simulink model "manual_steer_19b"  (R2019b)
settings: Solver=ode4  StartTime=0.0  StopTime=100  RelTol=1e-3
model workspace (MAT data in the model file):
  x2xx = 0
values from neighbouring files (symbols this model uses):
  KDspd = 0    [time_validation.m]
  KIspd = 0    [time_validation.m]
  KPspd = 20    [time_validation.m]
  PARSa = [ ... (first row only)    [Q_ART_par.m]
  PARSu = zeros(Nu,5)    [Q_ART_par.m]
  TOTALMASS = sum (M,'all')    [Q_ART_par.m]
  v_ref = vconst    (= 5.55555555556)    [time_validation.m]
undefined symbols (not defined in the file or in its folder): axle_rate_limit, BRAKE, brake_lag, brake_rate, DRIVE, Lspd, Nspd, Q0, QD0, RW, Tb, Tmc, Tst, Uspd
libraries: CarMaker4SL x72, simulink x5, TruckMaker4SL x1
(part 2 of 5)

== system manual_steer_19b/truckmaker model/TruckMaker/IPG Vehicle/AFGc ==
  note: steering ratio
  Clock : Clock
  Constant2 : Constant  Value=v_ref
  Constant3 : Constant  Value=PARSa
  From Workspace : FromWorkspace  VariableName=[tstr_in,str_in]  SampleTime=-1
  Gain1 : Gain  Gain=1/20
  MATLAB Function : MATLAB Function  TreatAsAtomicUnit=on
  Rate Limiter1 : RateLimiter  RisingSlewLimit=axle_rate_limit  FallingSlewLimit=-axle_rate_limit  SampleTimeMode=inherited
  To Workspace1 : ToWorkspace  VariableName=time  SampleTime=-1
  brake and drive controller : Subsystem
  find_vx : MATLAB Function  TreatAsAtomicUnit=on
  proc : Subsystem
  q&qd builder : Subsystem
  speed controller : Subsystem
  steering controller : Subsystem
  tractor brake : Outport
  wires:
  speed controller/1(accel command) -> brake and drive controller/1(acc command)
  brake and drive controller/1(tractor brake) -> tractor brake/1
  Rate Limiter1/1 -> steering controller/1(steer6)
  Constant3/1 -> MATLAB Function/2(PARSa)
  Gain1/1 -> MATLAB Function/1(str1)
  MATLAB Function/1(y) -> Rate Limiter1/1
  From Workspace/1 -> Gain1/1
  [q_truckmaker] -> find_vx/1(q)
  find_vx/1(vx6) -> speed controller/2(vxa)
  [qd_truckmaker] -> find_vx/2(qd)
  Constant2/1 -> speed controller/1(speed ref)
  Clock/1 -> To Workspace1/1

== system manual_steer_19b/truckmaker model/TruckMaker/IPG Vehicle/Brake ==
  note: <Your model here>
  note: When replacing the entire braking system,
      | be sure to disable the IPG brake model by using the brake
      | model 'Model Manager off' in the vehicle GUI.
  Sync_In : Inport
  Brake.IF.In : Inport  Port=2
  VhclCtrl.Brake : Inport  Port=3
  tractor brake : Inport  Port=4
  Brake : S-Function  FunctionName=TM_Sfun  Parameters='Brake'  SFunctionDeploymentMode=off  EnableBusSupport=off
  BrakeUpd : S-Function  FunctionName=TM_Sfun  Parameters='BrakeUpd'  SFunctionDeploymentMode=off  EnableBusSupport=off
  BusCreator : BusCreator  Inputs=32
  CreateBus Vhcl.Wheel.PT : Subsystem
  Demux : Demux  Outputs=32
      settings: DisplayOption=none
  Demux1 : Demux  Outputs=3
  Terminator{,1..5} (6 alike) : Terminator
  Sync_Out : Outport
  Vhcl.Wheel.PT : Outport  Port=2
  wires:
  Demux/32 -> BusCreator/32  "Brake IF Trq_DriveSrc_trg d7"
  Demux/31 -> BusCreator/31  "Brake IF Trq_DriveSrc_trg d6"
  Demux/30 -> BusCreator/30  "Brake IF Trq_DriveSrc_trg d5"
  Demux/29 -> BusCreator/29  "Brake IF Trq_DriveSrc_trg d4"
  Demux/28 -> BusCreator/28  "Brake IF Trq_DriveSrc_trg d3"
  Demux/27 -> BusCreator/27  "Brake IF Trq_DriveSrc_trg d2"
  Demux/26 -> BusCreator/26  "Brake IF Trq_DriveSrc_trg d1"
  Demux/25 -> BusCreator/25  "Brake IF Trq_DriveSrc_trg d0"
  Demux/24 -> BusCreator/24  "Brake IF Trq_Reg_trg FR2"
  Demux/23 -> BusCreator/23  "Brake IF Trq_Reg_trg FL2"
  Demux/22 -> BusCreator/22  "Brake IF Trq_Reg_trg RR2"
  Demux/21 -> BusCreator/21  "Brake IF Trq_Reg_trg RL2"
  Demux/20 -> BusCreator/20  "Brake IF Trq_Reg_trg RR"
  Demux/19 -> BusCreator/19  "Brake IF Trq_Reg_trg RL"
  Demux/18 -> BusCreator/18  "Brake IF Trq_Reg_trg FR"
  Demux/17 -> BusCreator/17  "Brake IF Trq_Reg_trg FL"
  Demux/16 -> BusCreator/16  "Brake IF Trq_PB FR2"
  Demux/15 -> BusCreator/15  "Brake IF Trq_PB FL2"
  Demux/14 -> BusCreator/14  "Brake IF Trq_PB RR2"
  Demux/13 -> BusCreator/13  "Brake IF Trq_PB RL2"
  Demux/12 -> BusCreator/12  "Brake IF Trq_PB RR"
  Demux/11 -> BusCreator/11  "Brake IF Trq_PB RL"
  Demux/10 -> BusCreator/10  "Brake IF Trq_PB FR"
  Demux/9 -> BusCreator/9  "Brake IF Trq_PB FL"
  Demux/8 -> BusCreator/8  "Brake IF Trq_WB FR2"
  Demux/7 -> BusCreator/7  "Brake IF Trq_WB FL2"
  BusCreator/1 -> BrakeUpd/2
  Brake/2 -> Demux/1
  BrakeUpd/1 -> Sync_Out/1
  Brake/1 -> BrakeUpd/1  "Sync"
  Brake.IF.In/1 -> Brake/2
  VhclCtrl.Brake/1 -> Brake/3
  Sync_In/1 -> Brake/1
  BrakeUpd/2 -> CreateBus Vhcl.Wheel.PT/1(In)
  CreateBus Vhcl.Wheel.PT/1(Out) -> Vhcl.Wheel.PT/1
  Demux1/2 -> BusCreator/3, BusCreator/4
  Demux1/1 -> BusCreator/1, BusCreator/2
  tractor brake/1 -> Demux1/1
  Demux/4 -> Terminator3/1  "Brake IF Trq_WB RR"
  Demux/3 -> Terminator2/1  "Brake IF Trq_WB RL"
  Demux/2 -> Terminator1/1  "Brake IF Trq_WB FR"
  Demux/1 -> Terminator/1  "Brake IF Trq_WB FL"
  Demux/5 -> Terminator4/1  "Brake IF Trq_WB RL2"
  Demux/6 -> Terminator5/1  "Brake IF Trq_WB RR2"
  Demux1/3 -> BusCreator/5, BusCreator/6

== system manual_steer_19b/truckmaker model/TruckMaker/IPG Vehicle/CarAndTrailer ==
  Sync_In : Inport
  VhclCtrl.Steering : Inport  Port=2
  Vhcl.Wheel.In : Inport  Port=3
  Vhcl.Misc : Inport  Port=4
  CarAndTrailerUpd : Subsystem
  Forces : Subsystem
  Ground : Ground
  Kinematics : Subsystem
  Kinetics : Subsystem
  Steering : Subsystem
  Terminator : Terminator
  Terminator1 : Terminator
  Trailer : Subsystem
  Sync_Out : Outport
  Brake.IF.In : Outport  Port=2
  wires:
  Ground/1 -> CarAndTrailerUpd/14(Vhcl.Fr1A)
  Trailer/13(Car.Hitch.FrcTrq) -> CarAndTrailerUpd/13(Car.Hitch.FrcTrq)
  Trailer/12(Vhcl.Wheel.FR2) -> CarAndTrailerUpd/12(Vhcl.Wheel.FR2)
  Trailer/11(Vhcl.Wheel.FL2) -> CarAndTrailerUpd/11(Vhcl.Wheel.FL2)
  Trailer/10(Vhcl.Wheel.RR2) -> CarAndTrailerUpd/10(Vhcl.Wheel.RR2)
  Trailer/9(Vhcl.Wheel.RL2) -> CarAndTrailerUpd/9(Vhcl.Wheel.RL2)
  Trailer/8(Vhcl.Wheel.RR) -> CarAndTrailerUpd/8(Vhcl.Wheel.RR)
  Trailer/7(Vhcl.Wheel.RL) -> CarAndTrailerUpd/7(Vhcl.Wheel.RL)
  Trailer/6(Vhcl.Wheel.FR) -> CarAndTrailerUpd/6(Vhcl.Wheel.FR)
  Trailer/5(Vhcl.Wheel.FL) -> CarAndTrailerUpd/5(Vhcl.Wheel.FL)
  Trailer/4(Vhcl.PoI) -> CarAndTrailerUpd/4(Vhcl.PoI)
  Trailer/3(Vhcl.Motion) -> CarAndTrailerUpd/3(Vhcl.Motion)
  Trailer/2(Vhcl.Steering) -> CarAndTrailerUpd/2(Vhcl.Steering)
  Trailer/1(Sync_Out) -> CarAndTrailerUpd/1(Sync_In)
  CarAndTrailerUpd/2(Brake.IF.In) -> Brake.IF.In/1
  Vhcl.Misc/1 -> Terminator1/1
  Vhcl.Wheel.In/1 -> Terminator/1
  Kinetics/6(WheelCarrier.Misc) -> Trailer/6(WheelCarrier.Misc)
  Kinetics/5(Car.Trq_T2W) -> Trailer/5(Car.Trq_T2W)
  Steering/2(Steer.IF) -> Kinematics/2(Steer.IF)
  Kinetics/4(Car.Fr1) -> Trailer/4(Car.Fr1)
  Kinetics/3(Car.Hitch) -> Trailer/3(Car.Hitch)
  Kinetics/2(Trailer.Load) -> Trailer/2(Trailer.Load)
  VhclCtrl.Steering/1 -> Steering/2(VhclCtrl.Steering)
  Sync_In/1 -> Steering/1(Sync_In)
  Steering/1(Sync_Out) -> Kinematics/1(Sync_In)
  Kinetics/1(Sync_Out) -> Trailer/1(Sync_In)
  Kinematics/5(lBuf) -> Forces/5(lBuf)
  Forces/8(FBuf_ext) -> Kinetics/8(FBuf_ext)
  Forces/4(Car.Load) -> Kinetics/4(Car.Load)
  Forces/7(FStabi_ext) -> Kinetics/7(FStabi_ext)
  Forces/6(FDamp_ext) -> Kinetics/6(FDamp_ext)
  Forces/5(FSpring_ext) -> Kinetics/5(FSpring_ext)
  Forces/2(Car.Virtual) -> Kinetics/2(Car.Virtual)
  Kinematics/2(lSpring) -> Forces/2(lSpring)
  Kinematics/3(vDamp) -> Forces/3(vDamp)
  Forces/3(Car.Aero) -> Kinetics/3(Car.Aero)
  Forces/1(Sync_Out) -> Kinetics/1(Sync_In)
  Kinematics/1(Sync_Out) -> Forces/1(Sync_In)
  Kinematics/4(lStabi) -> Forces/4(lStabi)
  CarAndTrailerUpd/1(Sync_Out) -> Sync_Out/1

== system manual_steer_19b/truckmaker model/TruckMaker/IPG Vehicle/PowerTrain ==
  note: When replacing the entire powertrain,
      | be sure to disable the IPG powertrain model by using the powertrain
      | model 'Model Manager off' in the vehicle GUI.
  note: <Your model here>
  Sync_In : Inport
  Vhcl.Wheel.PT : Inport  Port=2
  VhclCtrl.PT : Inport  Port=3
  BusCreator : BusCreator  Inputs=70
  Demux : Demux  Outputs=70
      settings: DisplayOption=none
  PowerTrain : S-Function  FunctionName=TM_Sfun  Parameters='PowerTrain'  SFunctionDeploymentMode=off  EnableBusSupport=off
  PowerTrainUpd : S-Function  FunctionName=TM_Sfun  Parameters='PowerTrainUpd'  SFunctionDeploymentMode=off  EnableBusSupport=off
  Sync_Out : Outport
  wires:
  Demux/70 -> BusCreator/70  "PT IF WFR2 Trq_BrakeReg_max"
  Demux/69 -> BusCreator/69  "PT IF WFR2 Trq_BrakeReg"
  Demux/68 -> BusCreator/68  "PT IF WFR2 Trq_Supp2WC"
  Demux/67 -> BusCreator/67  "PT IF WFR2 Trq_Drive"
  Demux/66 -> BusCreator/66  "PT IF WFR2 Trq_B2W"
  Demux/65 -> BusCreator/65  "PT IF WFR2 rotv"
  Demux/64 -> BusCreator/64  "PT IF WFR2 rot"
  Demux/63 -> BusCreator/63  "PT IF WFL2 Trq_BrakeReg_max"
  Demux/62 -> BusCreator/62  "PT IF WFL2 Trq_BrakeReg"
  Demux/59 -> BusCreator/59  "PT IF WFL2 Trq_B2W"
  Demux/58 -> BusCreator/58  "PT IF WFL2 rotv"
  Demux/57 -> BusCreator/57  "PT IF WFL2 rot"
  Demux/56 -> BusCreator/56  "PT IF WRR2 Trq_BrakeReg_max"
  Demux/55 -> BusCreator/55  "PT IF WRR2 Trq_BrakeReg"
  Demux/52 -> BusCreator/52  "PT IF WRR2 Trq_B2W"
  Demux/51 -> BusCreator/51  "PT IF WRR2 rotv"
  Demux/50 -> BusCreator/50  "PT IF WRR2 rot"
  Demux/49 -> BusCreator/49  "PT IF WRL2 Trq_BrakeReg_max"
  Demux/48 -> BusCreator/48  "PT IF WRL2 Trq_BrakeReg"
  Demux/45 -> BusCreator/45  "PT IF WRL2 Trq_B2W"
  Demux/44 -> BusCreator/44  "PT IF WRL2 rotv"
  Demux/43 -> BusCreator/43  "PT IF WRL2 rot"
  Demux/42 -> BusCreator/42  "PT IF WRR Trq_BrakeReg_max"
  Demux/41 -> BusCreator/41  "PT IF WRR Trq_BrakeReg"
  Demux/38 -> BusCreator/38  "PT IF WRR Trq_B2W"
  Demux/37 -> BusCreator/37  "PT IF WRR rotv"
  Demux/36 -> BusCreator/36  "PT IF WRR rot"
  Demux/35 -> BusCreator/35  "PT IF WRL Trq_BrakeReg_max"
  Demux/34 -> BusCreator/34  "PT IF WRL Trq_BrakeReg"
  Demux/31 -> BusCreator/31  "PT IF WRL Trq_B2W"
  Demux/30 -> BusCreator/30  "PT IF WRL rotv"
  Demux/29 -> BusCreator/29  "PT IF WRL rot"
  Demux/28 -> BusCreator/28  "PT IF WFR Trq_BrakeReg_max"
  Demux/27 -> BusCreator/27  "PT IF WFR Trq_BrakeReg"
  Demux/24 -> BusCreator/24  "PT IF WFR Trq_B2W"
  Demux/23 -> BusCreator/23  "PT IF WFR rotv"
  Demux/22 -> BusCreator/22  "PT IF WFR rot"
  Demux/21 -> BusCreator/21  "PT IF WFL Trq_BrakeReg_max"
  Demux/20 -> BusCreator/20  "PT IF WFL Trq_BrakeReg"
  Demux/17 -> BusCreator/17  "PT IF WFL Trq_B2W"
  Demux/16 -> BusCreator/16  "PT IF WFL rotv"
  Demux/15 -> BusCreator/15  "PT IF WFL rot"
  Demux/14 -> BusCreator/14  "PT IF DL_iDiff_mean"
  Demux/13 -> BusCreator/13  "PT IF Trq_Supp2BdyEng y"
  Demux/12 -> BusCreator/12  "PT IF Trq_Supp2BdyEng x"
  Demux/11 -> BusCreator/11  "PT IF Trq_Supp2Bdy1B z"
  Demux/10 -> BusCreator/10  "PT IF Trq_Supp2Bdy1B y"
  Demux/9 -> BusCreator/9  "PT IF Trq_Supp2Bdy1B x"
  Demux/8 -> BusCreator/8  "PT IF Trq_Supp2Bdy1 z"
  Demux/7 -> BusCreator/7  "PT IF Trq_Supp2Bdy1 y"
  Demux/6 -> BusCreator/6  "PT IF Trq_Supp2Bdy1 x"
  Demux/5 -> BusCreator/5  "PT IF Engine_rotv"
  Demux/4 -> BusCreator/4  "PT IF GearNo"
  Demux/3 -> BusCreator/3  "PT IF OperationError"
  Demux/2 -> BusCreator/2  "PT IF OperationState"
  Demux/1 -> BusCreator/1  "PT IF Ignition"
  BusCreator/1 -> PowerTrainUpd/2
  PowerTrain/2 -> Demux/1
  Sync_In/1 -> PowerTrain/1
  PowerTrainUpd/1 -> Sync_Out/1
  PowerTrain/1 -> PowerTrainUpd/1  "Sync"
  VhclCtrl.PT/1 -> PowerTrain/3
  Vhcl.Wheel.PT/1 -> PowerTrain/2
  Demux/60 -> BusCreator/60  "PT IF WFL2 Trq_Drive"
  Demux/61 -> BusCreator/61  "PT IF WFL2 Trq_Supp2WC"
  Demux/18 -> BusCreator/18  "PT IF WFL Trq_Drive"
  Demux/19 -> BusCreator/19  "PT IF WFL Trq_Supp2WC"
  Demux/25 -> BusCreator/25  "PT IF WFR Trq_Drive"
  Demux/26 -> BusCreator/26  "PT IF WFR Trq_Supp2WC"
  Demux/32 -> BusCreator/32  "PT IF WRL Trq_Drive"
  Demux/33 -> BusCreator/33  "PT IF WRL Trq_Supp2WC"
  Demux/39 -> BusCreator/39  "PT IF WRR Trq_Drive"
  Demux/40 -> BusCreator/40  "PT IF WRR Trq_Supp2WC"
  Demux/46 -> BusCreator/46  "PT IF WRL2 Trq_Drive"
  Demux/47 -> BusCreator/47  "PT IF WRL2 Trq_Supp2WC"
  Demux/53 -> BusCreator/53  "PT IF WRR2 Trq_Drive"
  Demux/54 -> BusCreator/54  "PT IF WRR2 Trq_Supp2WC"

== system manual_steer_19b/truckmaker model/TruckMaker/VehicleControl/CreateBus Vhcl.Misc ==
  In1 : Inport
  Bus Creator5 : BusCreator  Inputs=11
  Demux5 : Demux  Outputs=11
      settings: DisplayOption=none
  Out1 : Outport
  wires:
  Demux5/11 -> Bus Creator5/11  "Vhcl Wind_vel_0 z"
  Demux5/10 -> Bus Creator5/10  "Vhcl Wind_vel_0 y"
  Demux5/9 -> Bus Creator5/9  "Vhcl Wind_vel_0 x"
  Demux5/8 -> Bus Creator5/8  "Vhcl DL2BdyEng y"
  Demux5/7 -> Bus Creator5/7  "Vhcl DL2BdyEng x"
  Demux5/6 -> Bus Creator5/6  "Vhcl TrqDL2Bdy1B z"
  Demux5/5 -> Bus Creator5/5  "Vhcl TrqDL2Bdy1B y"
  Demux5/4 -> Bus Creator5/4  "Vhcl TrqDL2Bdy1B x"
  Demux5/3 -> Bus Creator5/3  "Vhcl Trq_DL2Bdy1 z"
  In1/1 -> Demux5/1
  Bus Creator5/1 -> Out1/1
  Demux5/2 -> Bus Creator5/2  "Vhcl Trq_DL2Bdy1 y"
  Demux5/1 -> Bus Creator5/1  "Vhcl Trq_DL2Bdy1 x"

== system manual_steer_19b/truckmaker model/TruckMaker/VehicleControl/CreateBus Vhcl.Wheel.In ==
  In1 : Inport
  Bus Creator1 : BusCreator  Inputs=24
  Demux1 : Demux  Outputs=24
      settings: DisplayOption=none
  Out1 : Outport
  wires:
  Demux1/12 -> Bus Creator1/12  "Vhcl Wheel RR rotv"
  Demux1/11 -> Bus Creator1/11  "Vhcl Wheel RR Trq_DL2WC"
  Demux1/10 -> Bus Creator1/10  "Vhcl Wheel RR Trq_B2WC"
  Demux1/9 -> Bus Creator1/9  "Vhcl Wheel RL rotv"
  Demux1/8 -> Bus Creator1/8  "Vhcl Wheel RL Trq_DL2WC"
  Demux1/7 -> Bus Creator1/7  "Vhcl Wheel RL Trq_B2WC"
  Demux1/6 -> Bus Creator1/6  "Vhcl Wheel FR rotv"
  Demux1/5 -> Bus Creator1/5  "Vhcl Wheel FR Trq_DL2WC"
  Demux1/4 -> Bus Creator1/4  "Vhcl Wheel FR Trq_B2WC"
  Demux1/3 -> Bus Creator1/3  "Vhcl Wheel FL rotv"
  Demux1/2 -> Bus Creator1/2  "Vhcl Wheel FL Trq_DL2WC"
  Demux1/1 -> Bus Creator1/1  "Vhcl Wheel FL Trq_B2WC"
  Bus Creator1/1 -> Out1/1
  In1/1 -> Demux1/1
  Demux1/24 -> Bus Creator1/24  "Vhcl Wheel FR2 rotv"
  Demux1/23 -> Bus Creator1/23  "Vhcl Wheel FR2 Trq_DL2WC"
  Demux1/22 -> Bus Creator1/22  "Vhcl Wheel FR2 Trq_B2WC"
  Demux1/21 -> Bus Creator1/21  "Vhcl Wheel FL2 rotv"
  Demux1/20 -> Bus Creator1/20  "Vhcl Wheel FL2 Trq_DL2WC"
  Demux1/19 -> Bus Creator1/19  "Vhcl Wheel FL2 Trq_B2WC"
  Demux1/18 -> Bus Creator1/18  "Vhcl Wheel RR2 rotv"
  Demux1/17 -> Bus Creator1/17  "Vhcl Wheel RR2 Trq_DL2WC"
  Demux1/16 -> Bus Creator1/16  "Vhcl Wheel RR2 Trq_B2WC"
  Demux1/15 -> Bus Creator1/15  "Vhcl Wheel RL2 rotv"
  Demux1/14 -> Bus Creator1/14  "Vhcl Wheel RL2 Trq_DL2WC"
  Demux1/13 -> Bus Creator1/13  "Vhcl Wheel RL2 Trq_B2WC"

== system manual_steer_19b/truckmaker model/TruckMaker/VehicleControl/CreateBus VhclCtrl ==
  In : Inport
  BusCreator : BusCreator  Inputs=29
  Demux : Demux  Outputs=29
      settings: DisplayOption=none
  Out : Outport
  wires:
  Demux/29 -> BusCreator/29  "VhclCtrl Lights Reverse"
  Demux/28 -> BusCreator/28  "VhclCtrl Lights Brake"
  Demux/27 -> BusCreator/27  "VhclCtrl Lights FogRear"
  Demux/26 -> BusCreator/26  "VhclCtrl Lights FogFrontR"
  Demux/25 -> BusCreator/25  "VhclCtrl Lights FogFrontL"
  Demux/24 -> BusCreator/24  "VhclCtrl Lights IndR"
  Demux/23 -> BusCreator/23  "VhclCtrl Lights IndL"
  Demux/22 -> BusCreator/22  "VhclCtrl Lights ParkR"
  Demux/21 -> BusCreator/21  "VhclCtrl Lights ParkL"
  Demux/20 -> BusCreator/20  "VhclCtrl Lights Daytime"
  Demux/19 -> BusCreator/19  "VhclCtrl Lights HighBeam"
  Demux/18 -> BusCreator/18  "VhclCtrl Lights LowBeam"
  Demux/17 -> BusCreator/17  "VhclCtrl Steering Trq"
  Demux/16 -> BusCreator/16  "VhclCtrl Steering AngAcc"
  Demux/15 -> BusCreator/15  "VhclCtrl Steering AngVel"
  Demux/14 -> BusCreator/14  "VhclCtrl Steering Ang"
  Demux/13 -> BusCreator/13  "VhclCtrl Gas"
  Demux/12 -> BusCreator/12  "VhclCtrl Clutch"
  Demux/11 -> BusCreator/11  "VhclCtrl BrakePark"
  Demux/10 -> BusCreator/10  "VhclCtrl Brake"
  Demux/9 -> BusCreator/9  "VhclCtrl SelectorCtrl"
  Demux/8 -> BusCreator/8  "VhclCtrl GearNo"
  Demux/7 -> BusCreator/7  "VhclCtrl UserSignal4"
  Demux/6 -> BusCreator/6  "VhclCtrl UserSignal3"
  Demux/5 -> BusCreator/5  "VhclCtrl UserSignal2"
  Demux/4 -> BusCreator/4  "VhclCtrl UserSignal1"
  Demux/3 -> BusCreator/3  "VhclCtrl UserSignal0"
  Demux/2 -> BusCreator/2  "VhclCtrl Key"
  Demux/1 -> BusCreator/1  "VhclCtrl SST"
  BusCreator/1 -> Out/1
  In/1 -> Demux/1

== system manual_steer_19b/truckmaker model/TruckMaker/VehicleControl/CreateBus VhclCtrl.PT ==
  In1 : Inport
  BusCreator1 : BusCreator  Inputs=12
  Demux1 : Demux  Outputs=12
      settings: DisplayOption=none
  Out1 : Outport
  wires:
  BusCreator1/1 -> Out1/1
  In1/1 -> Demux1/1
  Demux1/1 -> BusCreator1/1  "VhclCtrl SST"
  Demux1/2 -> BusCreator1/2  "VhclCtrl Key"
  Demux1/3 -> BusCreator1/3  "VhclCtrl UserSignal0"
  Demux1/4 -> BusCreator1/4  "VhclCtrl UserSignal1"
  Demux1/5 -> BusCreator1/5  "VhclCtrl UserSignal2"
  Demux1/6 -> BusCreator1/6  "VhclCtrl UserSignal3"
  Demux1/7 -> BusCreator1/7  "VhclCtrl UserSignal4"
  Demux1/8 -> BusCreator1/8  "VhclCtrl GearNo"
  Demux1/9 -> BusCreator1/9  "VhclCtrl SelectorCtrl"
  Demux1/10 -> BusCreator1/10  "VhclCtrl Clutch"
  Demux1/11 -> BusCreator1/11  "VhclCtrl Gas"
  Demux1/12 -> BusCreator1/12  "VhclCtrl Brake"

== system manual_steer_19b/truckmaker model/TruckMaker/VehicleControl/CreateBus VhclCtrl.Steering ==
  In1 : Inport
  Bus Creator : BusCreator  Inputs=5
  Demux : Demux  Outputs=5
      settings: DisplayOption=none
  Out1 : Outport
  wires:
  In1/1 -> Demux/1
  Bus Creator/1 -> Out1/1
  Demux/1 -> Bus Creator/1  "VhclCtrl Steering Ang"
  Demux/5 -> Bus Creator/5  "VhclCtrl Steering ByTrq"
  Demux/3 -> Bus Creator/3  "VhclCtrl Steering AngAcc"
  Demux/2 -> Bus Creator/2  "VhclCtrl Steering AngVel"
  Demux/4 -> Bus Creator/4  "VhclCtrl Steering Trq"

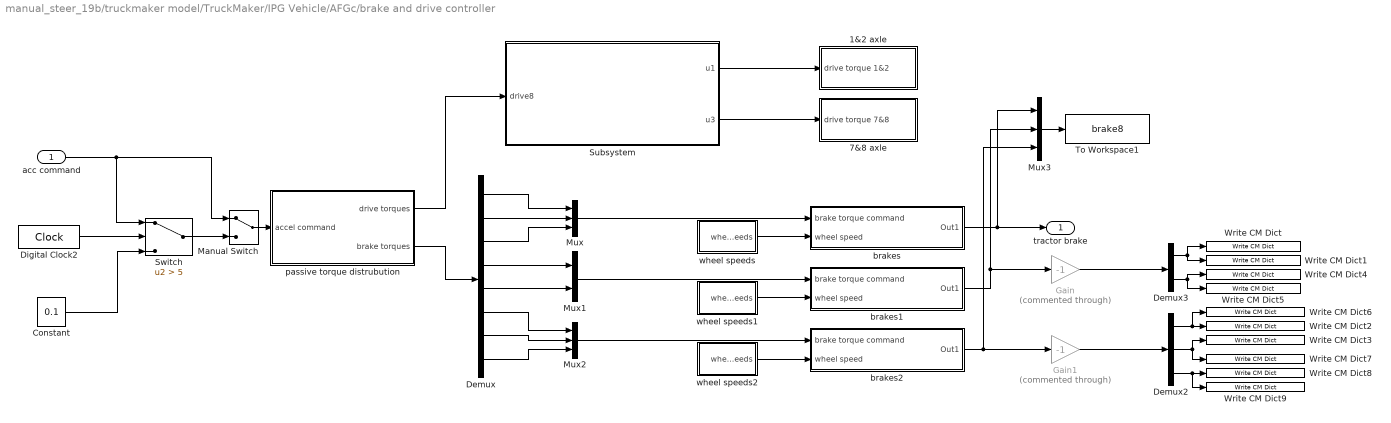
== system manual_steer_19b/truckmaker model/TruckMaker/IPG Vehicle/AFGc/brake and drive controller ==
  acc command : Inport
  1&2 axle : Subsystem
  7&8 axle : Subsystem
  Constant : Constant  Value=0.1
  Demux : Demux  Outputs=8
  Demux2 : Demux  Outputs=3
  Demux3 : Demux  Outputs=2
  Digital Clock2 : DigitalClock  SampleTime=0.001
  Gain : Gain  Commented=through  Gain=-1
  Gain1 : Gain  Commented=through  Gain=-1
  Manual Switch : ManualSwitch
  Mux : Mux  Inputs=3
  Mux1 : Mux  Inputs=2
  Mux2 : Mux  Inputs=3
  Mux3 : Mux  Inputs=3
  Subsystem : Subsystem
  Switch : Switch  Criteria=u2 > Threshold  Threshold=5
  To Workspace1 : ToWorkspace  VariableName=brake8  SampleTime=-1
  Write CM Dict : CarMaker4SL/Write CM Dict  xname=Tr.Brake.Trq_FL_ext  xsync=off
  Write CM Dict1 : CarMaker4SL/Write CM Dict  xname=Tr.Brake.Trq_FR_ext  xsync=off
  Write CM Dict2 : CarMaker4SL/Write CM Dict  xname=Tr2.Brake.Trq_FR_ext  xsync=off
  Write CM Dict3 : CarMaker4SL/Write CM Dict  xname=Tr2.Brake.Trq_ML_ext  xsync=off
  Write CM Dict4 : CarMaker4SL/Write CM Dict  xname=Tr.Brake.Trq_RL_ext  xsync=off
  Write CM Dict5 : CarMaker4SL/Write CM Dict  xname=Tr.Brake.Trq_RR_ext  xsync=off
  Write CM Dict6 : CarMaker4SL/Write CM Dict  xname=Tr2.Brake.Trq_FL_ext  xsync=off
  Write CM Dict7 : CarMaker4SL/Write CM Dict  xname=Tr2.Brake.Trq_MR_ext  xsync=off
  Write CM Dict8 : CarMaker4SL/Write CM Dict  xname=Tr2.Brake.Trq_RL_ext  xsync=off
  Write CM Dict9 : CarMaker4SL/Write CM Dict  xname=Tr2.Brake.Trq_RR_ext  xsync=off
  brakes : Subsystem
  brakes1 : Subsystem
  brakes2 : Subsystem
  passive torque distrubution : Subsystem
  wheel speeds : Subsystem
  wheel speeds1 : Subsystem
  wheel speeds2 : Subsystem
  tractor brake : Outport  VectorParamsAs1DForOutWhenUnconnected=off
  wires:
  passive torque distrubution/2(brake torques) -> Demux/1
  Mux/1 -> brakes/1(brake torque command)
  Mux1/1 -> brakes1/1(brake torque command)
  wheel speeds1/1(wheel speeds) -> brakes1/2(wheel speed)
  Mux2/1 -> brakes2/1(brake torque command)
  brakes/1(Out1) -> tractor brake/1, Mux3/1
  Mux3/1 -> To Workspace1/1
  Subsystem/1(u1) -> 1&2 axle/1(drive torque 1&2)
  Subsystem/2(u3) -> 7&8 axle/1(drive torque 7&8)
  wheel speeds2/1(wheel speeds) -> brakes2/2(wheel speed)
  wheel speeds/1(wheel speeds) -> brakes/2(wheel speed)
  Demux/1 -> Mux/1
  Demux/2 -> Mux/2
  Demux/3 -> Mux/3
  Demux/5 -> Mux1/2
  Demux/4 -> Mux1/1
  Demux/6 -> Mux2/1
  Demux/7 -> Mux2/2
  Demux/8 -> Mux2/3
  brakes1/1(Out1) -> Gain/1, Mux3/2
  Demux3/2 -> Write CM Dict4/1, Write CM Dict5/1
  Demux3/1 -> Write CM Dict/1, Write CM Dict1/1
  brakes2/1(Out1) -> Gain1/1, Mux3/3
  Demux2/1 -> Write CM Dict2/1, Write CM Dict6/1
  Demux2/2 -> Write CM Dict7/1, Write CM Dict3/1
  Demux2/3 -> Write CM Dict9/1, Write CM Dict8/1
  passive torque distrubution/1(drive torques) -> Subsystem/1(drive8)
  Gain/1 -> Demux3/1
  Gain1/1 -> Demux2/1
  acc command/1 -> Switch/1, Manual Switch/1
  Constant/1 -> Switch/3
  Digital Clock2/1 -> Switch/2
  Manual Switch/1 -> passive torque distrubution/1(accel command)
  Switch/1 -> Manual Switch/2

== system manual_steer_19b/truckmaker model/TruckMaker/IPG Vehicle/AFGc/proc ==
  Constant1 : Constant  Value=PARSu
  Constant2 : Constant  Value=PARSa
  MatMaker : MATLAB Function  TreatAsAtomicUnit=on
  To Workspace1 : ToWorkspace  Commented=on  VariableName=Va_out  SampleTime=-1
  To Workspace3 : ToWorkspace  Commented=on  VariableName=Vj_out  SampleTime=-1
  To Workspace5 : ToWorkspace  Commented=on  VariableName=Vg_out  SampleTime=-1
  To Workspace6 : ToWorkspace  VariableName=Vgg_out  SampleTime=-1
  To Workspace7 : ToWorkspace  Commented=on  VariableName=Vaa_out  SampleTime=-1
  wires:
  [qd_truckmaker] -> MatMaker/2(qd)
  MatMaker/1(Va) -> To Workspace1/1
  [q_truckmaker] -> MatMaker/1(q)
  MatMaker/5(Vgg) -> To Workspace6/1
  MatMaker/3(Vj) -> To Workspace3/1
  Constant1/1 -> MatMaker/3(PARSu)
  MatMaker/4(Vg) -> To Workspace5/1
  Constant2/1 -> MatMaker/4(PARSa)
  MatMaker/2(Vaa) -> To Workspace7/1

== system manual_steer_19b/truckmaker model/TruckMaker/IPG Vehicle/AFGc/q&qd builder ==
  Read CM Dict1 : CarMaker4SL/Read CM Dict  xname=Tr.ay  xsync=off  xstime=Continuous
  Read CM Dict2 : CarMaker4SL/Read CM Dict  xname=Tr2.ay  xsync=off  xstime=Continuous
  Read CM Dict3 : CarMaker4SL/Read CM Dict  xname=Car.ay  xsync=off  xstime=Continuous
  To Workspace : ToWorkspace  VariableName=q_out_truckmaker  SampleTime=-1
      settings: Save2DSignal=2-D array (concatenate along first dimension)
  To Workspace1 : ToWorkspace  VariableName=qd_out_truckmaker  SampleTime=-1
      settings: Save2DSignal=2-D array (concatenate along first dimension)
  To Workspace2 : ToWorkspace  VariableName=lat_acc_u1_out  SampleTime=-1
      settings: Save2DSignal=2-D array (concatenate along first dimension)
  To Workspace3 : ToWorkspace  VariableName=lat_acc_u2_out  SampleTime=-1
      settings: Save2DSignal=2-D array (concatenate along first dimension)
  To Workspace4 : ToWorkspace  VariableName=lat_acc_u3_out  SampleTime=-1
      settings: Save2DSignal=2-D array (concatenate along first dimension)
  build q : Subsystem
  build qd : Subsystem
  tag scope: q_truckmaker=global, qd_truckmaker=global
  wires:
  build q/1(q) -> To Workspace/1, [q_truckmaker]
  build qd/1(qd) -> To Workspace1/1, [qd_truckmaker]
  Read CM Dict3/1 -> To Workspace2/1
  Read CM Dict1/1 -> To Workspace3/1
  Read CM Dict2/1 -> To Workspace4/1

== system manual_steer_19b/truckmaker model/TruckMaker/IPG Vehicle/AFGc/speed controller ==
  speed ref : Inport
  vxa : Inport  Port=2
  PID Controller : simulink/Continuous/PID Controller  Controller=PID  Form=Parallel  TimeDomain=Discrete-time  SampleTime=-1  IntegratorMethod=Forward Euler  FilterMethod=Forward Euler  ControllerParametersSource=internal  P=KPspd  I=KIspd  D=KDspd  N=Nspd  UseFilter=on  TunerSelectOption=Transfer Function Based (PID Tuner App)  InitialConditionSource=internal  InitialConditionForIntegrator=0  InitialConditionForFilter=0  DifferentiatorICPrevScaledInput=0  ExternalReset=none  TrackingMode=off  Kt=1  LimitOutput=on  UpperSaturationLimit=Uspd  LowerSaturationLimit=Lspd  LinearizeAsGain=on  AntiWindupMode=clamping  Kb=1  POutMin=[]  POutMax=[]  IOutMin=[]  IOutMax=[]  DOutMin=[]  DOutMax=[]  NOutMin=[]  NOutMax=[]  SumOutMin=[]  SumOutMax=[]  SaturationOutMin=[]  SaturationOutMax=[]  PParamMin=[]  PParamMax=[]  IParamMin=[]  IParamMax=[]  DParamMin=[]  DParamMax=[]  NParamMin=[]  NParamMax=[]  KbParamMin=[]  KbParamMax=[]  KtParamMin=[]  KtParamMax=[]  KbOutMin=[]  KbOutMax=[]  KtOutMin=[]  KtOutMax=[]  IntegratorOutMin=[]  IntegratorOutMax=[]  FilterOutMin=[]  FilterOutMax=[]  SumI1OutMin=[]  SumI1OutMax=[]  SumI2OutMin=[]  SumI2OutMax=[]  SumI3OutMin=[]  SumI3OutMax=[]  SumI4OutMin=[]  SumI4OutMax=[]  SumDOutMin=[]  SumDOutMax=[]  DifferentiatorOutMin=[]  DifferentiatorOutMax=[]  FilterDiffOutCoefMin=[]  FilterDiffOutCoefMax=[]  ReciprocalOutMin=[]  ReciprocalOutMax=[]  SumDenOutMin=[]  SumDenOutMax=[]  SumNumOutMin=[]  SumNumOutMax=[]  DivideOutMin=[]  DivideOutMax=[]  IntegratorContinuousStateAttributes=''  IntegratorStateMustResolveToSignalObject=off  IntegratorRTWStateStorageClass=Auto  FilterContinuousStateAttributes=''  FilterStateMustResolveToSignalObject=off  FilterRTWStateStorageClass=Auto  ParallelPVariant=InternalParameters  IdealPVariant=Disabled  IVariant=InternalParameters  DVariant=InternalParameters  IntegratorVariant=Discrete  SatVariant=Enabled  AWVariant=DiscClampingParallel  PCopyVariant=Disabled  TRVariant=Disabled  FdbkBlocksVariant=Forward  IdealPFdbkVariant=Disabled  SatFdbkVariant=Disabled  DerivativeFilterVariant=ForwardEulerFilter  NVariant=InternalParameters  NCopyVariant=Disabled  FilterICVariant=InternalICsFilter  IntegratorICVariant=InternalICs  ExternalResetVariant=Disabled  TRSumVariant=Passthrough  SumFdbkVariant=Disabled  SumVariant=Sum_PID
  Sum : Sum  Inputs=|-+
  select U : Selector  InputPortWidth=6  IndexOptions=Index vector (dialog)  Indices=[1]  OutputSizes=1
  accel command : Outport
  wires:
  Sum/1 -> PID Controller/1
  vxa/1 -> select U/1
  select U/1 -> Sum/1
  speed ref/1 -> Sum/2
  PID Controller/1 -> accel command/1

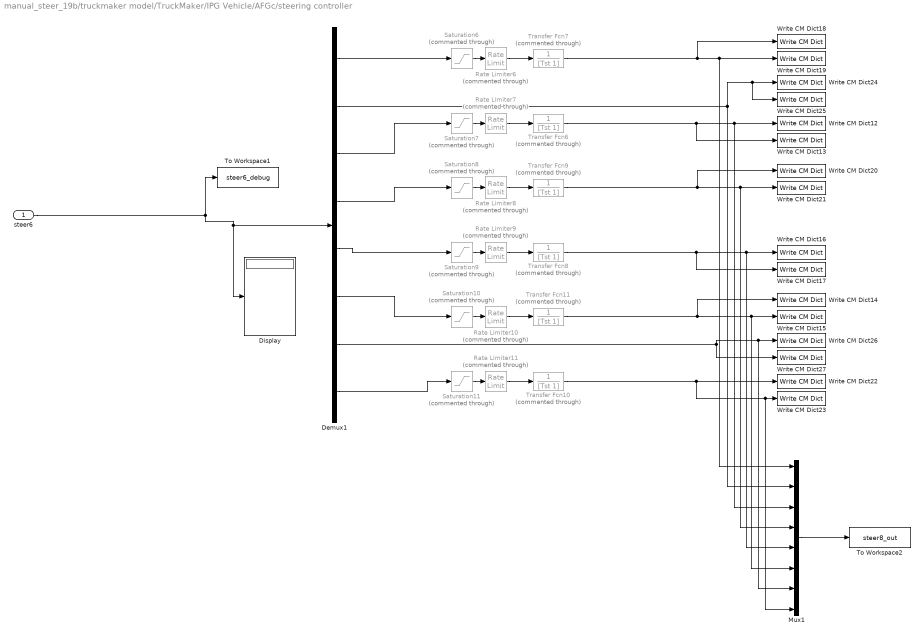
== system manual_steer_19b/truckmaker model/TruckMaker/IPG Vehicle/AFGc/steering controller ==
  steer6 : Inport
  Demux1 : Demux  Outputs=8
  Display : Display
  Mux1 : Mux  Inputs=8
  Rate Limiter{6..11} (6 alike) : RateLimiter  Commented=through  RisingSlewLimit=3  FallingSlewLimit=-3  SampleTimeMode=inherited
  Saturation10 : Saturate  Commented=through  UpperLimit=0.3491  LowerLimit=-0.3491
  Saturation11 : Saturate  Commented=through  UpperLimit=0.2443  LowerLimit=-0.2443
  Saturation6 : Saturate  Commented=through  UpperLimit=0.3491  LowerLimit=-0.3491
  Saturation7 : Saturate  Commented=through  UpperLimit=0.2443  LowerLimit=-0.2443
  Saturation8 : Saturate  Commented=through  UpperLimit=0.3491  LowerLimit=-0.3491
  Saturation9 : Saturate  Commented=through  UpperLimit=0.2443  LowerLimit=-0.2443
  To Workspace1 : ToWorkspace  VariableName=steer6_debug  SampleTime=-1
  To Workspace2 : ToWorkspace  VariableName=steer8_out  SampleTime=-1
  Transfer Fcn{6..11} (6 alike) : TransferFcn  Commented=through  Denominator=[Tst 1]
  Write CM Dict12 : CarMaker4SL/Write CM Dict  xname=Car.CRL2.rz_ext  xsync=off
  Write CM Dict13 : CarMaker4SL/Write CM Dict  xname=Car.CRR2.rz_ext  xsync=off
  Write CM Dict14 : CarMaker4SL/Write CM Dict  xname=Tr2.CFL.rz_ext  xsync=off
  Write CM Dict15 : CarMaker4SL/Write CM Dict  xname=Tr2.CFR.rz_ext  xsync=off
  Write CM Dict16 : CarMaker4SL/Write CM Dict  xname=Tr.CRL.rz_ext  xsync=off
  Write CM Dict17 : CarMaker4SL/Write CM Dict  xname=Tr.CRR.rz_ext  xsync=off
  Write CM Dict18 : CarMaker4SL/Write CM Dict  xname=Car.CFL.rz_ext  xsync=off
  Write CM Dict19 : CarMaker4SL/Write CM Dict  xname=Car.CFR.rz_ext  xsync=off
  Write CM Dict20 : CarMaker4SL/Write CM Dict  xname=Tr.CFL.rz_ext  xsync=off
  Write CM Dict21 : CarMaker4SL/Write CM Dict  xname=Tr.CFR.rz_ext  xsync=off
  Write CM Dict22 : CarMaker4SL/Write CM Dict  xname=Tr2.CRL.rz_ext  xsync=off
  Write CM Dict23 : CarMaker4SL/Write CM Dict  xname=Tr2.CRR.rz_ext  xsync=off
  Write CM Dict24 : CarMaker4SL/Write CM Dict  xname=Car.CRL.rz_ext  xsync=off
  Write CM Dict25 : CarMaker4SL/Write CM Dict  xname=Car.CRR.rz_ext  xsync=off
  Write CM Dict26 : CarMaker4SL/Write CM Dict  xname=Tr2.CML.rz_ext  xsync=off
  Write CM Dict27 : CarMaker4SL/Write CM Dict  xname=Tr2.CMR.rz_ext  xsync=off
  wires:
  Demux1/3 -> Saturation7/1
  Saturation8/1 -> Rate Limiter8/1
  Rate Limiter9/1 -> Transfer Fcn8/1
  Transfer Fcn8/1 -> Write CM Dict17/1, Mux1/5, Write CM Dict16/1
  Rate Limiter11/1 -> Transfer Fcn10/1
  Transfer Fcn9/1 -> Write CM Dict20/1, Mux1/4, Write CM Dict21/1
  Demux1/5 -> Saturation9/1
  Demux1/1 -> Saturation6/1
  Transfer Fcn7/1 -> Write CM Dict18/1, Mux1/1, Write CM Dict19/1
  Saturation9/1 -> Rate Limiter9/1
  Saturation10/1 -> Rate Limiter10/1
  Rate Limiter7/1 -> Transfer Fcn6/1
  Demux1/6 -> Saturation10/1
  Rate Limiter10/1 -> Transfer Fcn11/1
  Rate Limiter6/1 -> Transfer Fcn7/1
  Saturation6/1 -> Rate Limiter6/1
  Saturation7/1 -> Rate Limiter7/1
  Demux1/4 -> Saturation8/1
  Saturation11/1 -> Rate Limiter11/1
  Demux1/8 -> Saturation11/1
  Transfer Fcn11/1 -> Write CM Dict14/1, Mux1/6, Write CM Dict15/1
  Transfer Fcn6/1 -> Write CM Dict13/1, Mux1/3, Write CM Dict12/1
  Rate Limiter8/1 -> Transfer Fcn9/1
  Transfer Fcn10/1 -> Mux1/8, Write CM Dict23/1, Write CM Dict22/1
  Demux1/7 -> Mux1/7, Write CM Dict26/1, Write CM Dict27/1
  Demux1/2 -> Write CM Dict25/1, Write CM Dict24/1, Mux1/2
  Mux1/1 -> To Workspace2/1
  steer6/1 -> Display/1, Demux1/1, To Workspace1/1

== system manual_steer_19b/truckmaker model/TruckMaker/IPG Vehicle/Brake/CreateBus Vhcl.Wheel.PT ==
  In : Inport
  BusCreator : BusCreator  Inputs=40
  Demux : Demux  Outputs=40
      settings: DisplayOption=none
  Out : Outport
  wires:
  Demux/40 -> BusCreator/40  "Vhcl Trq_DriveSrc_trg d7"
  Demux/39 -> BusCreator/39  "Vhcl Trq_DriveSrc_trg d6"
  Demux/38 -> BusCreator/38  "Vhcl Trq_DriveSrc_trg d5"
  Demux/37 -> BusCreator/37  "Vhcl Trq_DriveSrc_trg d4"
  Demux/36 -> BusCreator/36  "Vhcl Trq_DriveSrc_trg d3"
  Demux/35 -> BusCreator/35  "Vhcl Trq_DriveSrc_trg d2"
  Demux/34 -> BusCreator/34  "Vhcl Trq_DriveSrc_trg d1"
  Demux/33 -> BusCreator/33  "Vhcl Trq_DriveSrc_trg d0"
  Demux/32 -> BusCreator/32  "Vhcl Wheel FR2 WhlBearing"
  Demux/31 -> BusCreator/31  "Vhcl Wheel FR2 Trq_T2W"
  Demux/30 -> BusCreator/30  "Vhcl Wheel FR2 Trq_BrakeReg_trg"
  Demux/29 -> BusCreator/29  "Vhcl Wheel FR2 Trq_Brake"
  Demux/28 -> BusCreator/28  "Vhcl Wheel FL2 WhlBearing"
  Demux/27 -> BusCreator/27  "Vhcl Wheel FL2 Trq_T2W"
  Demux/26 -> BusCreator/26  "Vhcl Wheel FL2 Trq_BrakeReg_trg"
  Demux/25 -> BusCreator/25  "Vhcl Wheel FL2 Trq_Brake"
  Demux/24 -> BusCreator/24  "Vhcl Wheel RR2 WhlBearing"
  Demux/23 -> BusCreator/23  "Vhcl Wheel RR2 Trq_T2W"
  Demux/22 -> BusCreator/22  "Vhcl Wheel RR2 Trq_BrakeReg_trg"
  Demux/21 -> BusCreator/21  "Vhcl Wheel RR2 Trq_Brake"
  Demux/20 -> BusCreator/20  "Vhcl Wheel RL2 WhlBearing"
  Demux/19 -> BusCreator/19  "Vhcl Wheel RL2 Trq_T2W"
  Demux/18 -> BusCreator/18  "Vhcl Wheel RL2 Trq_BrakeReg_trg"
  Demux/17 -> BusCreator/17  "Vhcl Wheel RL2 Trq_Brake"
  Demux/16 -> BusCreator/16  "Vhcl Wheel RR WhlBearing"
  Demux/15 -> BusCreator/15  "Vhcl Wheel RR Trq_T2W"
  Demux/14 -> BusCreator/14  "Vhcl Wheel RR Trq_BrakeReg_trg"
  Demux/13 -> BusCreator/13  "Vhcl Wheel RR Trq_Brake"
  Demux/12 -> BusCreator/12  "Vhcl Wheel RL WhlBearing"
  Demux/11 -> BusCreator/11  "Vhcl Wheel RL Trq_T2W"
  Demux/10 -> BusCreator/10  "Vhcl Wheel RL Trq_BrakeReg_trg"
  Demux/9 -> BusCreator/9  "Vhcl Wheel RL Trq_Brake"
  Demux/8 -> BusCreator/8  "Vhcl Wheel FR WhlBearing"
  Demux/7 -> BusCreator/7  "Vhcl Wheel FR Trq_T2W"
  Demux/6 -> BusCreator/6  "Vhcl Wheel FR Trq_BrakeReg_trg"
  Demux/5 -> BusCreator/5  "Vhcl Wheel FR Trq_Brake"
  Demux/4 -> BusCreator/4  "Vhcl Wheel FL WhlBearing"
  Demux/3 -> BusCreator/3  "Vhcl Wheel FL Trq_T2W"
  Demux/2 -> BusCreator/2  "Vhcl Wheel FL Trq_BrakeReg_trg"
  Demux/1 -> BusCreator/1  "Vhcl Wheel FL Trq_Brake"
  BusCreator/1 -> Out/1
  In/1 -> Demux/1

== system manual_steer_19b/truckmaker model/TruckMaker/IPG Vehicle/CarAndTrailer/CarAndTrailerUpd ==
  Sync_In : Inport
  Vhcl.Steering : Inport  Port=2
  Vhcl.Motion : Inport  Port=3
  Vhcl.PoI : Inport  Port=4
  Vhcl.Wheel.FL : Inport  Port=5
  Vhcl.Wheel.FR : Inport  Port=6
  Vhcl.Wheel.RL : Inport  Port=7
  Vhcl.Wheel.RR : Inport  Port=8
  Vhcl.Wheel.RL2 : Inport  Port=9
  Vhcl.Wheel.RR2 : Inport  Port=10
  Vhcl.Wheel.FL2 : Inport  Port=11
  Vhcl.Wheel.FR2 : Inport  Port=12
  Car.Hitch.FrcTrq : Inport  Port=13
  Vhcl.Fr1A : Inport  Port=14
  CarAndTrailerUpd : S-Function  FunctionName=TM_Sfun  Parameters='CarAndTrUpd'  SFunctionDeploymentMode=off  EnableBusSupport=off
  CreateBus Brake.IF.In : Subsystem
  Sync_Out : Outport
  Brake.IF.In : Outport  Port=2
  wires:
  Vhcl.Fr1A/1 -> CarAndTrailerUpd/14  "user vehicle only"
  Vhcl.Wheel.RL2/1 -> CarAndTrailerUpd/9
  Vhcl.Wheel.RR2/1 -> CarAndTrailerUpd/10
  Vhcl.Wheel.FL2/1 -> CarAndTrailerUpd/11
  Vhcl.Wheel.FR2/1 -> CarAndTrailerUpd/12
  Car.Hitch.FrcTrq/1 -> CarAndTrailerUpd/13
  Vhcl.Wheel.RR/1 -> CarAndTrailerUpd/8
  Vhcl.Wheel.RL/1 -> CarAndTrailerUpd/7
  Vhcl.Wheel.FR/1 -> CarAndTrailerUpd/6
  Vhcl.Wheel.FL/1 -> CarAndTrailerUpd/5
  Vhcl.Steering/1 -> CarAndTrailerUpd/2
  Vhcl.Motion/1 -> CarAndTrailerUpd/3
  Vhcl.PoI/1 -> CarAndTrailerUpd/4
  CarAndTrailerUpd/2 -> CreateBus Brake.IF.In/1(In)
  CreateBus Brake.IF.In/1(Out) -> Brake.IF.In/1
  CarAndTrailerUpd/1 -> Sync_Out/1
  Sync_In/1 -> CarAndTrailerUpd/1

== system manual_steer_19b/truckmaker model/TruckMaker/IPG Vehicle/CarAndTrailer/Forces ==
  Sync_In : Inport
  lSpring : Inport  Port=2
  vDamp : Inport  Port=3
  lStabi : Inport  Port=4
  lBuf : Inport  Port=5
  External Suspension Forces : Subsystem
  Suspension Forces : Subsystem
  Vehicle Forces : Subsystem
  Sync_Out : Outport
  Car.Virtual : Outport  Port=2
  Car.Aero : Outport  Port=3
  Car.Load : Outport  Port=4
  FSpring_ext : Outport  Port=5
  FDamp_ext : Outport  Port=6
  FStabi_ext : Outport  Port=7
  FBuf_ext : Outport  Port=8
  wires:
  Sync_In/1 -> External Suspension Forces/1(Sync_In), Vehicle Forces/1(Sync_In)
  Vehicle Forces/2(Car.Virtual) -> Car.Virtual/1
  Vehicle Forces/3(Car.Aero) -> Car.Aero/1
  Vehicle Forces/4(Car.Load) -> Car.Load/1
  lSpring/1 -> Suspension Forces/2(lSpring), External Suspension Forces/2(lSpring)
  External Suspension Forces/2(FDamp_ext) -> FDamp_ext/1
  vDamp/1 -> Suspension Forces/3(vDamp), External Suspension Forces/3(vDamp)
  lStabi/1 -> Suspension Forces/4(lStabi), External Suspension Forces/4(lStabi)
  External Suspension Forces/3(FStabi_ext) -> FStabi_ext/1
  External Suspension Forces/1(FSpring_ext) -> FSpring_ext/1
  lBuf/1 -> Suspension Forces/5(lBuf), External Suspension Forces/5(lBuf)
  External Suspension Forces/4(FBuf_ext) -> FBuf_ext/1
  Vehicle Forces/1(Sync_Out) -> Suspension Forces/1(Sync_In)
  Suspension Forces/1(Sync_Out) -> Sync_Out/1

== system manual_steer_19b/truckmaker model/TruckMaker/IPG Vehicle/CarAndTrailer/Kinematics ==
  Sync_In : Inport
  Steer.IF : Inport  Port=2
  Kinematics : S-Function  FunctionName=TM_Sfun  Parameters='Kinematics'  SFunctionDeploymentMode=off  EnableBusSupport=off
  TireFL.In : Terminator
  TireFR.In : Terminator
  TireRL.In : Terminator
  TireRR.In : Terminator
  Sync_Out : Outport
  lSpring : Outport  Port=2
  vDamp : Outport  Port=3
  lStabi : Outport  Port=4
  lBuf : Outport  Port=5
  wires:
  Kinematics/8 -> lStabi/1
  Kinematics/2 -> TireFL.In/1
  Kinematics/3 -> TireFR.In/1
  Kinematics/4 -> TireRL.In/1
  Kinematics/5 -> TireRR.In/1
  Kinematics/6 -> lSpring/1
  Kinematics/7 -> vDamp/1
  Sync_In/1 -> Kinematics/1
  Kinematics/1 -> Sync_Out/1
  Steer.IF/1 -> Kinematics/2
  Kinematics/9 -> lBuf/1

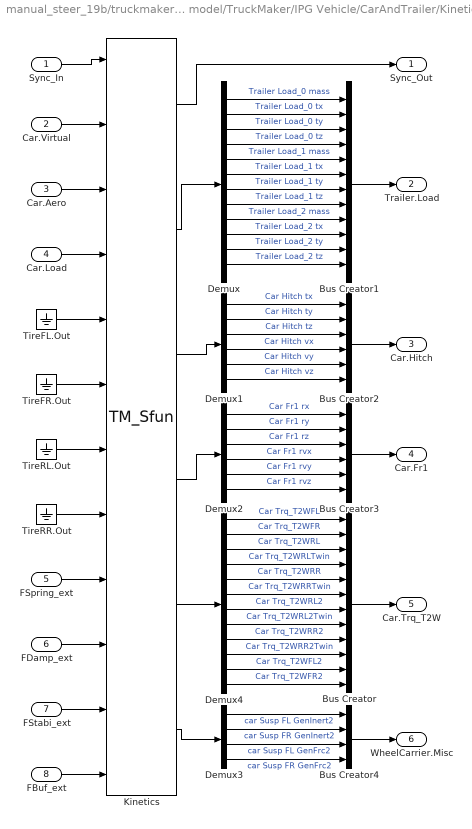
== system manual_steer_19b/truckmaker model/TruckMaker/IPG Vehicle/CarAndTrailer/Kinetics ==
  Sync_In : Inport
  Car.Virtual : Inport  Port=2
  Car.Aero : Inport  Port=3
  Car.Load : Inport  Port=4
  FSpring_ext : Inport  Port=5
  FDamp_ext : Inport  Port=6
  FStabi_ext : Inport  Port=7
  FBuf_ext : Inport  Port=8
  Bus Creator : BusCreator  Inputs=12
  Bus Creator1 : BusCreator  Inputs=12
  Bus Creator2 : BusCreator  Inputs=6
  Bus Creator3 : BusCreator  Inputs=6
  Bus Creator4 : BusCreator  Inputs=4
  Demux : Demux  Outputs=12
      settings: DisplayOption=none
  Demux1 : Demux  Outputs=6
      settings: DisplayOption=none
  Demux2 : Demux  Outputs=6
      settings: DisplayOption=none
  Demux3 : Demux
      settings: DisplayOption=none
  Demux4 : Demux  Outputs=12
      settings: DisplayOption=none
  Kinetics : S-Function  FunctionName=TM_Sfun  Parameters='Kinetics'  SFunctionDeploymentMode=off  EnableBusSupport=off
  TireFL.Out : Ground
  TireFR.Out : Ground
  TireRL.Out : Ground
  TireRR.Out : Ground
  Sync_Out : Outport
  Trailer.Load : Outport  Port=2
  Car.Hitch : Outport  Port=3
  Car.Fr1 : Outport  Port=4
  Car.Trq_T2W : Outport  Port=5
  WheelCarrier.Misc : Outport  Port=6
  wires:
  Demux4/12 -> Bus Creator/12  "Car Trq_T2WFR2"
  Demux4/11 -> Bus Creator/11  "Car Trq_T2WFL2"
  Sync_In/1 -> Kinetics/1
  Kinetics/1 -> Sync_Out/1
  Car.Aero/1 -> Kinetics/3
  Car.Virtual/1 -> Kinetics/2
  Bus Creator1/1 -> Trailer.Load/1
  Demux/1 -> Bus Creator1/1  "Trailer Load_0 mass"
  Demux/2 -> Bus Creator1/2  "Trailer Load_0 tx"
  Demux/3 -> Bus Creator1/3  "Trailer Load_0 ty"
  Demux/4 -> Bus Creator1/4  "Trailer Load_0 tz"
  Kinetics/2 -> Demux/1
  Demux/5 -> Bus Creator1/5  "Trailer Load_1 mass"
  Demux/6 -> Bus Creator1/6  "Trailer Load_1 tx"
  Demux/7 -> Bus Creator1/7  "Trailer Load_1 ty"
  Demux/8 -> Bus Creator1/8  "Trailer Load_1 tz"
  Demux/9 -> Bus Creator1/9  "Trailer Load_2 mass"
  Demux/10 -> Bus Creator1/10  "Trailer Load_2 tx"
  Demux/11 -> Bus Creator1/11  "Trailer Load_2 ty"
  Demux/12 -> Bus Creator1/12  "Trailer Load_2 tz"
  Demux1/1 -> Bus Creator2/1  "Car Hitch tx"
  Demux1/2 -> Bus Creator2/2  "Car Hitch ty"
  Demux1/3 -> Bus Creator2/3  "Car Hitch tz"
  Demux1/4 -> Bus Creator2/4  "Car Hitch vx"
  Demux1/5 -> Bus Creator2/5  "Car Hitch vy"
  Demux1/6 -> Bus Creator2/6  "Car Hitch vz"
  Kinetics/3 -> Demux1/1
  Bus Creator2/1 -> Car.Hitch/1
  Demux2/1 -> Bus Creator3/1  "Car Fr1 rx"
  Demux2/2 -> Bus Creator3/2  "Car Fr1 ry"
  Demux2/3 -> Bus Creator3/3  "Car Fr1 rz"
  Demux2/4 -> Bus Creator3/4  "Car Fr1 rvx"
  Demux2/5 -> Bus Creator3/5  "Car Fr1 rvy"
  Demux2/6 -> Bus Creator3/6  "Car Fr1 rvz"
  Bus Creator3/1 -> Car.Fr1/1
  Kinetics/4 -> Demux2/1
  Car.Load/1 -> Kinetics/4
  Demux3/1 -> Bus Creator4/1  "car Susp FL GenInert2"
  Demux3/2 -> Bus Creator4/2  "car Susp FR GenInert2"
  Demux3/3 -> Bus Creator4/3  "car Susp FL GenFrc2"
  Demux3/4 -> Bus Creator4/4  "car Susp FR GenFrc2"
  Bus Creator4/1 -> WheelCarrier.Misc/1
  Demux4/3 -> Bus Creator/3  "Car Trq_T2WRL"
  Demux4/2 -> Bus Creator/2  "Car Trq_T2WFR"
  Demux4/1 -> Bus Creator/1  "Car Trq_T2WFL"
  TireFL.Out/1 -> Kinetics/5
  TireFR.Out/1 -> Kinetics/6
  TireRL.Out/1 -> Kinetics/7
  TireRR.Out/1 -> Kinetics/8
  FSpring_ext/1 -> Kinetics/9
  FDamp_ext/1 -> Kinetics/10
  FStabi_ext/1 -> Kinetics/11
  Kinetics/6 -> Demux3/1
  Kinetics/5 -> Demux4/1
  Bus Creator/1 -> Car.Trq_T2W/1
  Demux4/9 -> Bus Creator/9  "Car Trq_T2WRR2"
  Demux4/10 -> Bus Creator/10  "Car Trq_T2WRR2Twin"
  Demux4/7 -> Bus Creator/7  "Car Trq_T2WRL2"
  Demux4/8 -> Bus Creator/8  "Car Trq_T2WRL2Twin"
  Demux4/5 -> Bus Creator/5  "Car Trq_T2WRR"
  Demux4/4 -> Bus Creator/4  "Car Trq_T2WRLTwin"
  Demux4/6 -> Bus Creator/6  "Car Trq_T2WRRTwin"
  FBuf_ext/1 -> Kinetics/12

== system manual_steer_19b/truckmaker model/TruckMaker/IPG Vehicle/CarAndTrailer/Steering ==
  note: When replacing the entire steering system,
      | be sure to disable the IPG steering model by using the steering
      | model 'Model Manager off' in the vehicle GUI.
  Sync_In : Inport
  VhclCtrl.Steering : Inport  Port=2
  Bus Creator1 : BusCreator  Inputs=16
  Bus Creator2 : BusCreator  Inputs=5
  Demux : Demux  Outputs=21
      settings: DisplayOption=none
  Steering : S-Function  FunctionName=TM_Sfun  Parameters='Steering'  SFunctionDeploymentMode=off  EnableBusSupport=off
  Terminator : Terminator
  Sync_Out : Outport
  Steer.IF : Outport  Port=2
  wires:
  Demux/21 -> Bus Creator2/5  "Steering IF R Inert"
  Demux/20 -> Bus Creator2/4  "Steering IF R Frc"
  Demux/19 -> Bus Creator2/3  "Steering IF L Inert"
  Demux/18 -> Bus Creator2/2  "Steering IF L Frc"
  Demux/17 -> Bus Creator2/1  "Steering IF SteerByTrq"
  Demux/16 -> Bus Creator1/16  "Steering IF R iSteer2q"
  Demux/15 -> Bus Creator1/15  "Steering IF R qpp"
  Demux/14 -> Bus Creator1/14  "Steering IF R qp"
  Demux/13 -> Bus Creator1/13  "Steering IF R q"
  Demux/12 -> Bus Creator1/12  "Steering IF L iSteer2q"
  Demux/11 -> Bus Creator1/11  "Steering IF L qpp"
  Demux/10 -> Bus Creator1/10  "Steering IF L qp"
  Demux/9 -> Bus Creator1/9  "Steering IF L q"
  Demux/8 -> Bus Creator1/8  "Steering IF AssistTrqPin"
  Demux/7 -> Bus Creator1/7  "Steering IF AssistTrqCol"
  Demux/6 -> Bus Creator1/6  "Steering IF AssistFrc"
  Demux/5 -> Bus Creator1/5  "Steering IF TrqStatic"
  Demux/4 -> Bus Creator1/4  "Steering IF Trq"
  Demux/3 -> Bus Creator1/3  "Steering IF AngAcc"
  Demux/2 -> Bus Creator1/2  "Steering IF AngVel"
  Demux/1 -> Bus Creator1/1  "Steering IF Ang"
  Bus Creator1/1 -> Steer.IF/1
  Bus Creator2/1 -> Terminator/1  "Steer IF (in)"
  Sync_In/1 -> Steering/1
  Steering/1 -> Sync_Out/1
  VhclCtrl.Steering/1 -> Steering/2
  Steering/2 -> Demux/1

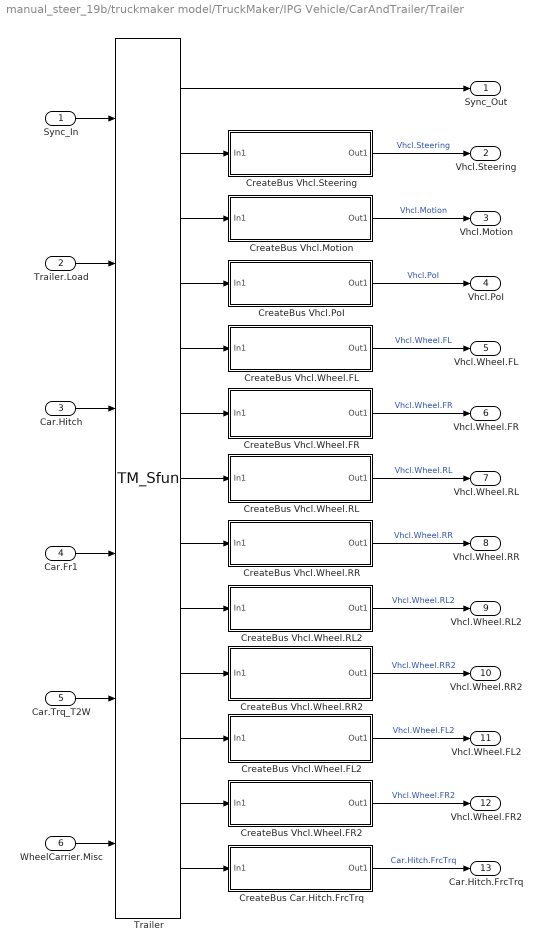
== system manual_steer_19b/truckmaker model/TruckMaker/IPG Vehicle/CarAndTrailer/Trailer ==
  Sync_In : Inport
  Trailer.Load : Inport  Port=2
  Car.Hitch : Inport  Port=3
  Car.Fr1 : Inport  Port=4
  Car.Trq_T2W : Inport  Port=5
  WheelCarrier.Misc : Inport  Port=6
  CreateBus Car.Hitch.FrcTrq : Subsystem
  CreateBus Vhcl.Motion : Subsystem
  CreateBus Vhcl.PoI : Subsystem
  CreateBus Vhcl.Steering : Subsystem
  CreateBus Vhcl.Wheel.FL : Subsystem
  CreateBus Vhcl.Wheel.FL2 : Subsystem
  CreateBus Vhcl.Wheel.FR : Subsystem
  CreateBus Vhcl.Wheel.FR2 : Subsystem
  CreateBus Vhcl.Wheel.RL : Subsystem
  CreateBus Vhcl.Wheel.RL2 : Subsystem
  CreateBus Vhcl.Wheel.RR : Subsystem
  CreateBus Vhcl.Wheel.RR2 : Subsystem
  Trailer : S-Function  FunctionName=TM_Sfun  Parameters='Trailer'  SFunctionDeploymentMode=off  EnableBusSupport=off
  Sync_Out : Outport
  Vhcl.Steering : Outport  Port=2
  Vhcl.Motion : Outport  Port=3
  Vhcl.PoI : Outport  Port=4
  Vhcl.Wheel.FL : Outport  Port=5
  Vhcl.Wheel.FR : Outport  Port=6
  Vhcl.Wheel.RL : Outport  Port=7
  Vhcl.Wheel.RR : Outport  Port=8
  Vhcl.Wheel.RL2 : Outport  Port=9
  Vhcl.Wheel.RR2 : Outport  Port=10
  Vhcl.Wheel.FL2 : Outport  Port=11
  Vhcl.Wheel.FR2 : Outport  Port=12
  Car.Hitch.FrcTrq : Outport  Port=13
  wires:
  CreateBus Vhcl.Wheel.RL2/1(Out1) -> Vhcl.Wheel.RL2/1  "Vhcl.Wheel.RL2"
  CreateBus Vhcl.Wheel.RR2/1(Out1) -> Vhcl.Wheel.RR2/1  "Vhcl.Wheel.RR2"
  CreateBus Vhcl.Wheel.FL2/1(Out1) -> Vhcl.Wheel.FL2/1  "Vhcl.Wheel.FL2"
  CreateBus Vhcl.Wheel.FR2/1(Out1) -> Vhcl.Wheel.FR2/1  "Vhcl.Wheel.FR2"
  Trailer/12 -> CreateBus Vhcl.Wheel.FR2/1(In1)
  Trailer/11 -> CreateBus Vhcl.Wheel.FL2/1(In1)
  Trailer/10 -> CreateBus Vhcl.Wheel.RR2/1(In1)
  Trailer/9 -> CreateBus Vhcl.Wheel.RL2/1(In1)
  CreateBus Vhcl.Wheel.FL/1(Out1) -> Vhcl.Wheel.FL/1  "Vhcl.Wheel.FL"
  CreateBus Vhcl.Wheel.FR/1(Out1) -> Vhcl.Wheel.FR/1  "Vhcl.Wheel.FR"
  CreateBus Vhcl.Wheel.RL/1(Out1) -> Vhcl.Wheel.RL/1  "Vhcl.Wheel.RL"
  CreateBus Vhcl.Wheel.RR/1(Out1) -> Vhcl.Wheel.RR/1  "Vhcl.Wheel.RR"
  Trailer/8 -> CreateBus Vhcl.Wheel.RR/1(In1)
  Trailer/7 -> CreateBus Vhcl.Wheel.RL/1(In1)
  Trailer/6 -> CreateBus Vhcl.Wheel.FR/1(In1)
  Trailer/5 -> CreateBus Vhcl.Wheel.FL/1(In1)
  Trailer/13 -> CreateBus Car.Hitch.FrcTrq/1(In1)
  Trailer/2 -> CreateBus Vhcl.Steering/1(In1)
  CreateBus Vhcl.Steering/1(Out1) -> Vhcl.Steering/1  "Vhcl.Steering"
  Trailer/3 -> CreateBus Vhcl.Motion/1(In1)
  Trailer/4 -> CreateBus Vhcl.PoI/1(In1)
  CreateBus Vhcl.PoI/1(Out1) -> Vhcl.PoI/1  "Vhcl.PoI"
  CreateBus Vhcl.Motion/1(Out1) -> Vhcl.Motion/1  "Vhcl.Motion"
  Car.Trq_T2W/1 -> Trailer/5
  WheelCarrier.Misc/1 -> Trailer/6
  CreateBus Car.Hitch.FrcTrq/1(Out1) -> Car.Hitch.FrcTrq/1  "Car.Hitch.FrcTrq"
  Car.Fr1/1 -> Trailer/4
  Car.Hitch/1 -> Trailer/3
  Trailer.Load/1 -> Trailer/2
  Trailer/1 -> Sync_Out/1
  Sync_In/1 -> Trailer/1

== system manual_steer_19b/truckmaker model/TruckMaker/IPG Vehicle/AFGc/brake and drive controller/1&2 axle ==
  drive torque 1&2 : Inport
  Constant2 : Constant  Value=0
  Gain{,1..3} (4 alike) : Gain  Gain=-1
  Gain4 : Gain  Commented=through  Gain=-1
  To Workspace : ToWorkspace  VariableName=drive_torque1  SampleTime=-1
  Write CM Dict : CarMaker4SL/Write CM Dict  xname=PT.WFL.Trq_Drive  xsync=off
  Write CM Dict1 : CarMaker4SL/Write CM Dict  xname=PT.WFR.Trq_Drive  xsync=off
  Write CM Dict2 : CarMaker4SL/Write CM Dict  xname=PT.WRL.Trq_Drive  xsync=off
  Write CM Dict3 : CarMaker4SL/Write CM Dict  xname=PT.WRR.Trq_Drive  xsync=off
  Write CM Dict4 : CarMaker4SL/Write CM Dict  xname=PT.WFL.Trq_Supp2WC  xsync=off
  Write CM Dict5 : CarMaker4SL/Write CM Dict  xname=PT.WFR.Trq_Supp2WC  xsync=off
  Write CM Dict6 : CarMaker4SL/Write CM Dict  xname=PT.WRL.Trq_Supp2WC  xsync=off
  Write CM Dict7 : CarMaker4SL/Write CM Dict  xname=PT.WRR.Trq_Supp2WC  xsync=off
  Write CM Dict8 : CarMaker4SL/Write CM Dict  xname=PT.Trq_Supp2Bdy1B.y  xsync=off
  Write CM Dict9 : CarMaker4SL/Write CM Dict  xname=PT.Trq_Supp2Bdy1.y  xsync=off
  wires:
  Gain/1 -> Write CM Dict4/1
  Gain1/1 -> Write CM Dict5/1
  Gain2/1 -> Write CM Dict6/1
  Constant2/1 -> Write CM Dict8/1, Write CM Dict9/1
  drive torque 1&2/1 -> Gain4/1
  Gain3/1 -> Write CM Dict7/1
  Gain4/1 -> Write CM Dict2/1, Gain2/1, Gain3/1, Write CM Dict3/1, To Workspace/1, Gain/1, Write CM Dict/1, Gain1/1, Write CM Dict1/1

== system manual_steer_19b/truckmaker model/TruckMaker/IPG Vehicle/AFGc/brake and drive controller/7&8 axle ==
  drive torque 7&8 : Inport
  Gain4 : Gain  Commented=through  Gain=-1
  Terminator : Terminator  Commented=on
  To Workspace : ToWorkspace  VariableName=drive_torque7_8  SampleTime=-1
  Write CM Dict1 : CarMaker4SL/Write CM Dict  xname=Tr2.Trq_Ext2WhlML  xsync=off
  Write CM Dict2 : CarMaker4SL/Write CM Dict  xname=Tr2.Trq_Ext2WhlRL  xsync=off
  Write CM Dict3 : CarMaker4SL/Write CM Dict  xname=Tr2.Trq_Ext2WhlRR  xsync=off
  Write CM Dict4 : CarMaker4SL/Write CM Dict  xname=Tr2.Trq_Ext2WhlMR  xsync=off
  wires:
  drive torque 7&8/1 -> Gain4/1, To Workspace/1
  Gain4/1 -> Write CM Dict1/1, Write CM Dict4/1, Write CM Dict3/1, Write CM Dict2/1

== system manual_steer_19b/truckmaker model/TruckMaker/IPG Vehicle/AFGc/brake and drive controller/Subsystem ==
  drive8 : Inport
  Demux1 : Demux  Outputs=8
  Mux : Mux  Inputs=8
  Rate Limiter : RateLimiter  Commented=through  RisingSlewLimit=500  FallingSlewLimit=-500  SampleTimeMode=inherited
  Rate Limiter1 : RateLimiter  Commented=through  RisingSlewLimit=500  FallingSlewLimit=-500  SampleTimeMode=inherited
  Saturation : Saturate  UpperLimit=1500  LowerLimit=0
  Saturation1 : Saturate  UpperLimit=1500  LowerLimit=0
  Terminator{,1..5} (6 alike) : Terminator
  To Workspace : ToWorkspace  VariableName=drive  SampleTime=-1
  Transfer Fcn1 : TransferFcn  Commented=through  Denominator=[Tst 1]
  Transfer Fcn2 : TransferFcn  Commented=through  Denominator=[Tst 1]
  u1 : Outport
  u3 : Outport  Port=2
  wires:
  Demux1/3 -> Terminator/1, Mux/3
  Demux1/8 -> Saturation1/1
  Demux1/4 -> Terminator1/1, Mux/4
  drive8/1 -> Demux1/1
  Demux1/7 -> Terminator5/1, Mux/7
  Transfer Fcn2/1 -> Mux/8, u3/1
  Demux1/2 -> Mux/2, Terminator4/1
  Saturation1/1 -> Rate Limiter1/1
  Transfer Fcn1/1 -> Mux/1, u1/1
  Saturation/1 -> Rate Limiter/1
  Demux1/5 -> Terminator2/1, Mux/5
  Mux/1 -> To Workspace/1
  Demux1/6 -> Terminator3/1, Mux/6
  Demux1/1 -> Saturation/1
  Rate Limiter1/1 -> Transfer Fcn2/1
  Rate Limiter/1 -> Transfer Fcn1/1

== system manual_steer_19b/truckmaker model/TruckMaker/IPG Vehicle/AFGc/brake and drive controller/brakes ==
  note: torque reverses if wheel goes backwards
  brake torque command : Inport
  wheel speed : Inport  Port=2
  Memory : Memory
  Product : Product
  Rate Limiter : RateLimiter  RisingSlewLimit=brake_rate  FallingSlewLimit=-brake_rate  SampleTimeMode=inherited
  Sign : Signum
  Transport Delay : TransportDelay  Commented=on  DelayTime=brake_lag
  first_order_lags : Subsystem  Commented=on
  Out1 : Outport  VectorParamsAs1DForOutWhenUnconnected=off
  wires:
  Sign/1 -> Product/2
  Product/1 -> Out1/1
  Memory/1 -> Sign/1
  wheel speed/1 -> Memory/1
  Rate Limiter/1 -> Product/1
  Transport Delay/1 -> first_order_lags/1(In1)
  brake torque command/1 -> Rate Limiter/1

== system manual_steer_19b/truckmaker model/TruckMaker/IPG Vehicle/AFGc/brake and drive controller/brakes1 ==
  note: torque reverses if wheel goes backwards
  brake torque command : Inport
  wheel speed : Inport  Port=2
  Memory : Memory
  Product : Product
  Rate Limiter : RateLimiter  RisingSlewLimit=brake_rate  FallingSlewLimit=-brake_rate  SampleTimeMode=inherited
  Sign : Signum
  Transport Delay : TransportDelay  Commented=on  DelayTime=brake_lag
  first_order_lags : Subsystem  Commented=on
  Out1 : Outport  VectorParamsAs1DForOutWhenUnconnected=off
  wires:
  Sign/1 -> Product/2
  Product/1 -> Out1/1
  Memory/1 -> Sign/1
  wheel speed/1 -> Memory/1
  Rate Limiter/1 -> Product/1
  Transport Delay/1 -> first_order_lags/1(In1)
  brake torque command/1 -> Rate Limiter/1
